simulink model "holidays2"  (R2020a)
settings: Solver=VariableStepAuto  StartTime=0.0  StopTime=10.0  RelTol=1e-3
libraries: commdigbbndam3 x2, commchan3 x1, commrandsrc3 x1, commsink2 x1, impairlib x1
settings Model: Creator=adi20  LastModifiedBy=adi20

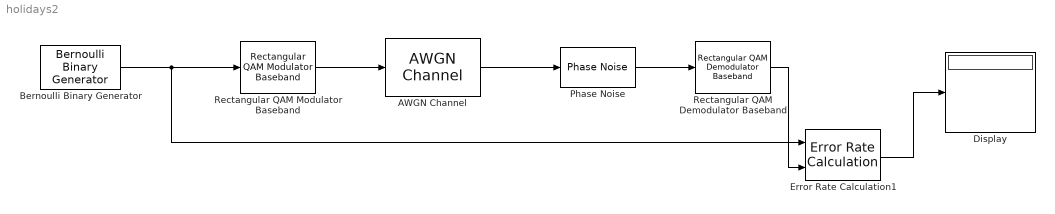
== system holidays2 ==
  AWGN Channel : commchan3/AWGN Channel  InputProcessing=Columns as channels (frame based)  seed=67  noiseMode="Signal to noise ratio  (Eb/No)"  EbNodB=20  EsNodB=10  SNRdB=10  bitsPerSym=8  Ps=1  Tsym=8*1e-4  variance=1
  Bernoulli Binary Generator : commrandsrc3/Bernoulli Binary Generator  ProbabilityOfZero=0.5  SeedSource=Auto  Seed=0  SampleTime=1e-4  SamplesPerFrame=8*250  OutputDataType=double  SimulateUsing=Interpreted execution
  Display : Display
  Error Rate Calculation1 : commsink2/Error Rate Calculation  N=0  st_delay=0  cp_mode=Entire frame  subframe=[]  PMode=Port  WsName=ErrorVec  RsMode2=off  stop=off  numErr=100  maxBits=1e6
  Phase Noise : impairlib/Phase Noise  Level=[ -60, -80 ]  FrequencyOffset=[ 20, 200 ]  SampleRate=1e4*8  RandomStream=mt19937ar with seed  Seed=2137  SimulateUsing=Interpreted execution
      settings: SourceProductBaseCode=CM,AM,SX
  Rectangular QAM Demodulator Baseband : commdigbbndam3/Rectangular QAM Demodulator Baseband  M=256  OutType=Bit  DecType=Hard decision  VarSource=Dialog  Variance=1  Dec=Binary  Mapping=[0:15]  PowType=Average Power  MinDist=2  AvgPow=1  PeakPow=1  Ph=0  outDtype1=Inherit via internal rule  outDtype2=Inherit via internal rule  derotateFactorWordLen=16  derotateFactorDataTypeStr=Inherit: Same word length as input  derotateFactorLastDataTypeStr=Inherit: Same word length as input  denormFactorWordLen=16  denormFactorDataTypeStr=Inherit: Same word length as input  denormFactorLastDataTypeStr=Inherit: Same word length as input  prodOutWordLen=32  prodOutOverflowMode=Wrap  prodOutRoundingMode=Floor  prodOutOvFlMode=off  prodOutOvFlModeLastStrValue=off  sumWordLen=32
  Rectangular QAM Modulator Baseband : commdigbbndam3/Rectangular QAM Modulator Baseband  M=256  InType=Bit  Enc=Binary  Mapping=[0:15]  PowType=Average Power  MinDist=2  AvgPow=1  PeakPow=1  Ph=0  outDtype=double  outWordLen=16  outUDDataType=sfix(16)  outFracLenMode=Best precision  outFracLen=15  outDataTypeStr=double  outLastDataTypeStr=double
  wires:
  Bernoulli Binary Generator/1 -> Error Rate Calculation1/1, Rectangular QAM Modulator Baseband/1
  Rectangular QAM Modulator Baseband/1 -> AWGN Channel/1
  AWGN Channel/1 -> Phase Noise/1
  Phase Noise/1 -> Rectangular QAM Demodulator Baseband/1
  Rectangular QAM Demodulator Baseband/1 -> Error Rate Calculation1/2
  Error Rate Calculation1/1 -> Display/1
